simulink library "xpcobsoletelib"  (Simulink 6.0)
settings: Solver=ode45  SolverMode=SingleTasking  StartTime=0.0  StopTime=10.0  RelTol=1e-3
values from neighbouring files (symbols this model uses):
  channels = round(channels)    [mbwaudpmc.m]
undefined symbols (not defined in the file or in its folder): mdiobvmpmcdio64, menccbcioquad
settings Model: Creator=adowd  LastModifiedBy=adowd
settings DataIOCC: SignalLoggingName=logsOut
settings OptimizationCC: BooleanDataType=off
settings DebuggingCC: CheckExecutionContextPreStartOutputMsg=on  CheckExecutionContextRuntimeOutputMsg=on  SolverPrmCheckMsg=none
settings HardwareCC: TargetUnknown=on
settings GRTTargetCC: UtilityFuncGeneration=Automatic  LifeSpan=inf
settings SFSimCC: SFSimApplyToAllLibs=on  SFSimBuildMode=Incremental

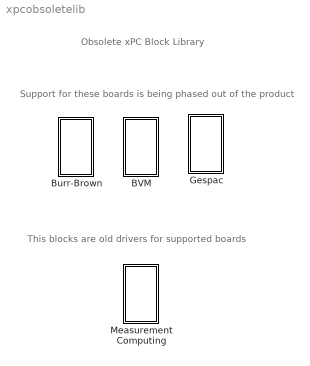
== system xpcobsoletelib ==
  note: Obsolete xPC Block Library
  note: Support for these boards is being phased out of the product
  note: This blocks are old drivers for supported boards
  BVM : Subsystem  EnableExecutionContextPropagation=on
  Burr-Brown : Subsystem  EnableExecutionContextPropagation=on
  Gespac : Subsystem  EnableExecutionContextPropagation=on
  Measurement Computing : Subsystem  EnableExecutionContextPropagation=on

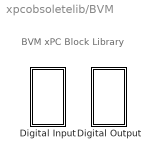
== system xpcobsoletelib/BVM ==
  note: BVM xPC Block Library
  Digital Input : Subsystem  EnableExecutionContextPropagation=on
  Digital Output : Subsystem  EnableExecutionContextPropagation=on

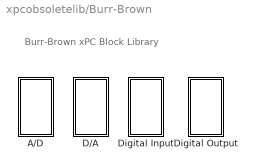
== system xpcobsoletelib/Burr-Brown ==
  note: Burr-Brown xPC Block Library
  A/D : Subsystem  EnableExecutionContextPropagation=on
  D/A : Subsystem  EnableExecutionContextPropagation=on
  Digital Input : Subsystem  EnableExecutionContextPropagation=on
  Digital Output : Subsystem  EnableExecutionContextPropagation=on

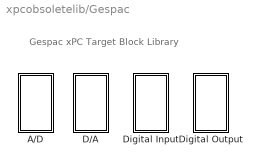
== system xpcobsoletelib/Gespac ==
  note: Gespac xPC Target Block Library
  A/D : Subsystem  EnableExecutionContextPropagation=on
  D/A : Subsystem  EnableExecutionContextPropagation=on
  Digital Input : Subsystem  EnableExecutionContextPropagation=on
  Digital Output : Subsystem  EnableExecutionContextPropagation=on

== system xpcobsoletelib/Measurement Computing ==
  note: Measurement Computing  xPC Target
      | Block Library (Obsolete)
  Incremental Encoder : Subsystem  EnableExecutionContextPropagation=on

== system xpcobsoletelib/BVM/Digital Input ==
  "PMCDIO64 " : S-Function  InitFcn=mdiobvmpmcdio64(1)  FunctionName=dibvmpmcdio64  Parameters=channel, port, ts, pcislot, config, fmt  mask(PMCDIO64-di){fmt=32 One bit channels, channel=[1], stopaction=, initial=, port=1, ts=0.001, pcislot=-1}
      mask prompts: fmt "Format:"; channel "Channel vector:"; port "Port (1-2):"; ts "Sample time:"; pcislot "PCI slot (-1: autosearch):"
      mask help:
      | PMCDIO64
      | BVM
      | Digital Input
      mask init:
      | [maskdisplay, maskdescription, config, initial, stopaction]=mdiobvmpmcdio64( 2, port, fmt, channel, stopaction, initial, pcislot); 
      | set_param(gcb,'MaskDisplay',maskdisplay);
      | set_param(gcb,'MaskDescription', maskdescription );
      mask Help: helpview(fullfile(docroot, 'mapfiles', 'xpc.map'), 'BVM_PMCDIO64_DIN')
      mask StyleString: popup(Single 32 bit port|32 One bit channels),edit,edit,edit,popup(1|2),edit,edit
      mask CallbackString:
      | maskvalues=get_param(gcb,'MaskValues');
      | 
      | fmt=maskvalues{1};
      | 
      | if fmt(1)=='3'
      | 
      | 	set_param(gcb, 'MaskEnables',{'on', 'on', 'off', 'off', 'on','on','on'});
      | 
      | else
      | 
      | 	set_param(gcb,'MaskEnables', {'on', 'off', 'off', 'off', 'on','on','on'});
      | 
      | end||||||
      mask Display: disp('PMCDIO64\nBVM\nDigital Input');port_label('output',1,'1');

== system xpcobsoletelib/BVM/Digital Output ==
  "PMCDIO64 1 " : S-Function  InitFcn=mdiobvmpmcdio64(1)  FunctionName=dobvmpmcdio64  Parameters=channel, port, ts, pcislot, config, fmt, stopaction, initial  mask(PMCDIO64-do){fmt=32 One bit channels, channel=[1], stopaction=[0], initial=[0], port=1, ts=0.001, pcislot=-1}
      mask prompts: fmt "Format:"; channel "Channel vector:"; stopaction "Reset action vector:"; initial "Initial value vector:"; port "Port (1-2):"; ts "Sample time:"; pcislot "PCI slot (-1: autosearch):"
      mask help:
      | PMCDIO64
      | BVM
      | Digital Output
      mask init:
      | [ maskdisplay, maskdescription, config, initial, stopaction ]=mdiobvmpmcdio64( 2, port, fmt, channel, stopaction, initial, pcislot);
      | set_param( gcb, 'MaskDisplay', maskdisplay );
      | set_param( gcb, 'MaskDescription', maskdescription );
      mask Help: helpview(fullfile(docroot, 'mapfiles', 'xpc.map'), 'BVM_PMCDIO64-1_DOUT')
      mask StyleString: popup(Single 32 bit port|32 One bit channels),edit,edit,edit,popup(1|2),edit,edit
      mask CallbackString:
      | maskvalues=get_param(gcb,'MaskValues');
      | 
      | fmt=maskvalues{1};
      | 
      | if fmt(1)=='3'
      | 
      | 	set_param(gcb, 'MaskEnables',{'on', 'on', 'on', 'on', 'on','on','on'});
      | 
      | else
      | 
      | 	set_param(gcb,'MaskEnables', {'on', 'off', 'on', 'on', 'on','on','on'});
      | 
      | end
      | 
      | ||||||
      mask Display: disp('PMCDIO64\nBVM\nDigital Output');port_label('input',1,'1');

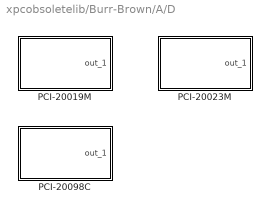
== system xpcobsoletelib/Burr-Brown/A/D ==
  "PCI-20019M " : Subsystem  EnableExecutionContextPropagation=on  mask(Analog Input Module){channels=1, range=-10, sampletime=0.001, module=1, baseaddress=0xd000}
      mask prompts: channels "Number of channels:"; range "Range vector:"; sampletime "Sample time:"; module "Module number (1-3):"; baseaddress "Base address (i.e. 0xd000):"
      mask help:
      | Burr-Brown
      | PCI-20019M
      | Analog Input
      mask init:
      | baseaddress=hex2dec(baseaddress(3:end));
      mask Help: helpview(fullfile(docroot, 'mapfiles', 'xpc.map'), 'Burr-Brown_PCI-20019M_AD')
      mask Display: disp('PCI-20019M\nBurr-Brown\nAnalog Input')
  "PCI-20023M " : Subsystem  EnableExecutionContextPropagation=on  mask(Analog Input Module){channels=1, range=-10, sampletime=0.001, module=1, baseaddress=0xd000}
      mask prompts: channels "Number of channels:"; range "Range vector:"; sampletime "Sample time:"; module "Module number (1-3):"; baseaddress "Base address (i.e. 0xd000):"
      mask help:
      | Burr-Brown
      | PCI-20023M
      | Analog Input
      mask init:
      | baseaddress=hex2dec(baseaddress(3:end));
      mask Help: helpview(fullfile(docroot, 'mapfiles', 'xpc.map'), 'Burr-Brown_PCI-20023M_AD')
      mask Display: disp('PCI-20023M\nBurr-Brown\nAnalog Input')
  "PCI-20098C " : Subsystem  EnableExecutionContextPropagation=on  mask(Analog Input Module){channels=1, range=+- 10 V, mux=Single-ended (16 channels), sampletime=0.001, baseaddress=0xd000}
      mask prompts: channels "Number of channels:"; range "Range vector:"; mux "Input coupling:"; sampletime "Sample time:"; baseaddress "Base address (i.e. 0xd000):"
      mask help:
      | Burr-Brown
      | PCI-20098C
      | Analog Input
      mask init:
      | baseaddress=hex2dec(baseaddress(3:end));
      mask Help: helpview(fullfile(docroot, 'mapfiles', 'xpc.map'), 'Burr-Brown_PCI-20098C_AD')
      mask StyleString: edit,popup(+- 10 V|+- 5V|0-10V),popup(Single-ended (16 channels)|Differential (8 channels)),edit,edit
      mask Display: disp('PCI-20098C\nBurr-Brown\nAnalog Input')

== system xpcobsoletelib/Burr-Brown/D/A ==
  "PCI-20003M " : Subsystem  EnableExecutionContextPropagation=on  mask(Analog Output Module){channels=[-10], sampletime=0.001, module=1, baseaddress=0xd000}
      mask prompts: channels "Channel vector:"; sampletime "Sample time:"; module "Module number (1-3):"; baseaddress "Base address (i.e. 0xd000):"
      mask help:
      | Burr-Brown
      | PCI-20003M
      | Analog Output
      mask init:
      | baseaddress=hex2dec(baseaddress(3:end));
      mask Help: helpview(fullfile(docroot, 'mapfiles', 'xpc.map'), 'Burr-Brown_PCI-20003M_DA')
      mask Display: disp('PCI-20003M\nBurr-Brown\nAnalog Output')

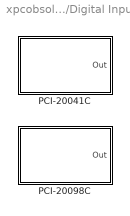
== system xpcobsoletelib/Burr-Brown/Digital Input ==
  "PCI-20041C " : Subsystem  EnableExecutionContextPropagation=on  mask(Digital Input Module){n_channels=1, port=0, sample_time=0.001, baseaddress=0xd000}
      mask prompts: n_channels "Number of channels:"; port "Port number (0-3):"; sample_time "Sample time:"; baseaddress "Base address (i.e. 0xd000):"
      mask help:
      | Burr Brown
      | PCI-20041C
      | Digital Input
      mask init:
      | baseaddress=hex2dec(baseaddress(3:end));
      mask Help: helpview(fullfile(docroot, 'mapfiles', 'xpc.map'), 'Burr-Brown_PCI-20041C_DIN')
      mask Display: disp('PCI-20041C\nBurr-Brown\nDigital Input')
  "PCI-20098C " : Subsystem  EnableExecutionContextPropagation=on  mask(Digital Input Module){n_channels=1, port=A, sample_time=0.001, baseaddress=0xd000}
      mask prompts: n_channels "Number of channels:"; sample_time "Sample time:"; baseaddress "Base address (i.e. 0xd000):"
      mask help:
      | Burr Brown
      | PCI-20098C
      | Digital Input
      mask init:
      | baseaddress=hex2dec(baseaddress(3:end));
      mask Help: helpview(fullfile(docroot, 'mapfiles', 'xpc.map'), 'Burr-Brown_PCI-20098C_DIN')
      mask StyleString: edit,popup(A|B),edit,edit
      mask Display: disp('PCI-20098C\nBurr-Brown\nDigital Input')

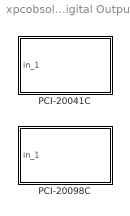
== system xpcobsoletelib/Burr-Brown/Digital Output ==
  "PCI-20041C " : Subsystem  EnableExecutionContextPropagation=on  mask(Digital Output Module){n_channels=1, port=0, sample_time=0.001, baseaddress=0xd000}
      mask prompts: n_channels "Number of channels:"; port "Port number (0-3):"; sample_time "Sample time:"; baseaddress "Base address (i.e. 0xd000):"
      mask help:
      | Burr Brown
      | PCI-20041C
      | Digital Output
      mask init:
      | baseaddress=hex2dec(baseaddress(3:end));
      mask Help: helpview(fullfile(docroot, 'mapfiles', 'xpc.map'), 'Burr-Brown_PCI-20041C_DOUT')
      mask Display: disp('PCI-20041C\nBurr-Brown\nDigital Output')
  "PCI-20098C " : Subsystem  EnableExecutionContextPropagation=on  mask(Digital Output Module){n_channels=1, port=A, sample_time=0.001, baseaddress=0xd000}
      mask prompts: n_channels "Number of channels:"; sample_time "Sample time:"; baseaddress "Base address (i.e. 0xd000):"
      mask help:
      | Burr Brown
      | PCI-20098C
      | Digital Output
      mask init:
      | baseaddress=hex2dec(baseaddress(3:end));
      mask Help: helpview(fullfile(docroot, 'mapfiles', 'xpc.map'), 'Burr-Brown_PCI-20098C_DOUT')
      mask StyleString: edit,popup(A|B),edit,edit
      mask Display: disp('PCI-20098C\nBurr-Brown\nDigital Output')

== system xpcobsoletelib/Gespac/A/D ==
  "GESADA-1 " : Subsystem  EnableExecutionContextPropagation=on  mask(Analog Input Module){channels=1, range=+-10 V, mux=Single-ended (16 channels), sampletime=0.001, baseaddress=0x300}
      mask prompts: channels "Number of channels:"; range "Range vector:"; mux "Input coupling:"; sampletime "Sample time:"; baseaddress "Base address (i.e. 0xd000):"
      mask help:
      | GESADA-1
      | Gespac
      | Analog Input
      mask init:
      | baseaddress=hex2dec(baseaddress(3:end));
      mask Help: helpview(fullfile(docroot, 'mapfiles', 'xpc.map'), 'Gespac_GESADA-1_AD')
      mask StyleString: edit,popup(+-10 V|+-5 V|0-10 V),popup(Single-ended (16 channels)|Differential (8 channels)),edit,edit
      mask Display: disp('GESADA-1\nGespac\nAnalog Input')

== system xpcobsoletelib/Gespac/D/A ==
  "GESADA-1 " : Subsystem  EnableExecutionContextPropagation=on  mask(Analog Output Module){channels=[-10], sampletime=0.001, baseaddress=0x300}
      mask prompts: channels "Channel vector:"; sampletime "Sample time:"; baseaddress "Base address (i.e. 0xd000):"
      mask help:
      | GESADA-1
      | Gespac
      | Analog Output
      mask init:
      | baseaddress=hex2dec(baseaddress(3:end));
      mask Help: helpview(fullfile(docroot, 'mapfiles', 'xpc.map'), 'Gespac_GESADA-1_DA')
      mask Display: disp('GESADA-1\nGespac\nAnalog Output')

== system xpcobsoletelib/Gespac/Digital Input ==
  "GESPIA-2A " : Subsystem  EnableExecutionContextPropagation=on  mask(Digital Input Module){n_channels=1, port=PIA0 A, sample_time=0.001, baseaddress=0x300}
      mask prompts: n_channels "Number of channels:"; port "Port name:"; sample_time "Sample time:"; baseaddress "Base address (i.e. 0xd000):"
      mask help:
      | Gespac
      | GESPIA-2A
      | Digital Input
      mask init:
      | baseaddress=hex2dec(baseaddress(3:end));
      mask Help: helpview(fullfile(docroot, 'mapfiles', 'xpc.map'), 'Gespac_GESPIA-2A_DIN')
      mask StyleString: edit,popup(PIA0 A|PIA0 B|PIA1 A|PIA1 B),edit,edit
      mask Display: disp('GESPIA-2A\nGespac\nDigital Input')

== system xpcobsoletelib/Gespac/Digital Output ==
  "GESPIA-2A " : Subsystem  EnableExecutionContextPropagation=on  mask(Digital Output Module){n_channels=1, port=PIA0 A, sample_time=0.001, baseaddress=0x300}
      mask prompts: n_channels "Number of channels:"; port "Port name:"; sample_time "Sample time:"; baseaddress "Base address (i.e. 0xd000):"
      mask help:
      | Gespac
      | GESPIA-2A
      | Digital Output
      mask init:
      | baseaddress=hex2dec(baseaddress(3:end));
      mask Help: helpview(fullfile(docroot, 'mapfiles', 'xpc.map'), 'Gespac_GESPIA-2A_DOUT')
      mask StyleString: edit,popup(PIA0 A|PIA0 B|PIA1 A|PIA1 B),edit,edit
      mask Display: disp('GESPIA-2A\nGespac\nDigital Output')

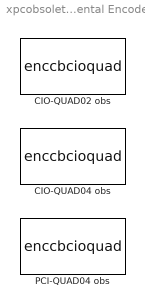
== system xpcobsoletelib/Measurement Computing/Incremental Encoder ==
  CIO-QUAD02 obs : S-Function  InitFcn=menccbcioquad(0);  FunctionName=enccbcioquad  Parameters=convBaseAddr, res, modetype, module, counting, rotation, prescale, ts, boardtype  mask(enccbcioquad){module=1, counting=Only First, rotation=Clockwise, modetype=single, res=1024, prescale=0, ts=0.001, baseAddr=0x300}
      mask prompts: module "Function module:"; counting "Counter reset by index:"; rotation "Positive rotation:"; modetype "Mode:"; res "Resolution:"; prescale "Filter prescale factor:"; ts "Sample time:"; baseAddr "Base address (i.e. 0xd000):"
      mask help:
      | CIO-QUAD02
      | Computer Boards
      | Incremental Encoder
      mask init:
      | convBaseAddr = 0;
      | boardtype = 1;
      | [convBaseAddr]=menccbcioquad(1, module ,baseAddr, 0, boardtype);
      mask Help: helpview(fullfile(docroot, 'mapfiles', 'xpc.map'), 'ComputerBoards_CIO-QUAD02_Encoder')
      mask StyleString: popup(1|2),popup(Continuous|Only first|Index input disabled),popup(Clockwise|Counter Clockwise),popup(Single|Double|Quadruple),edit,edit,edit,edit
      mask Display: text(0.05,0.75,'CIO-QUAD02','horizontalAlignment','left');text(0.05,0.5,'Comp. Boards','horizontalAlignment','left');text(0.05,0.25,'Inc. Encoder','horizontalAlignment','left');port_label('output',1,'Angle')port_label('output',2,'Turns')port_label('output',3,'Init')
  CIO-QUAD04 obs : S-Function  InitFcn=menccbcioquad(0);  FunctionName=enccbcioquad  Parameters=convBaseAddr, res, modetype, module, counting, rotation, prescale, ts, boardtype  mask(enccbcioquad){module=1, counting=Only first, rotation=Clockwise, modetype=Single, res=1024, prescale=0, ts=0.001, baseAddr=0x300}
      mask prompts: module "Function module:"; counting "Counting reset by index:"; rotation "Positive rotation:"; modetype "Mode:"; res "Resolution:"; prescale "Filter prescale factor:"; ts "Sample time:"; baseAddr "Base address (i.e. 0xd000):"
      mask help:
      | CIO-QUAD04
      | Computer Boards
      | Incremental Encoder
      mask init:
      | convBaseAddr = 0;
      | boardtype = 2;
      | [convBaseAddr]=menccbcioquad(1, module ,baseAddr, 0, boardtype);
      mask Help: helpview(fullfile(docroot, 'mapfiles', 'xpc.map'), 'ComputerBoards_CIO-QUAD04_Encoder')
      mask StyleString: popup(1|2|3|4),popup(Continuous|Only first|Index input disabled),popup(Clockwise|Counter Clockwise),popup(Single|Double|Quadruple),edit,edit,edit,edit
      mask Display: text(0.05,0.75,'CIO-QUAD04','horizontalAlignment','left');text(0.05,0.5,'Comp. Boards','horizontalAlignment','left');text(0.05,0.25,'Inc. Encoder','horizontalAlignment','left');port_label('output',1,'Angle')port_label('output',2,'Turns')port_label('output',3,'Init')
  PCI-QUAD04 obs : S-Function  InitFcn=menccbcioquad(0);  FunctionName=enccbcioquad  Parameters=convBaseAddr, res, modetype, module, counting, rotation, prescale, ts, boardtype  mask(enccbcioquad){module=1, counting=Only first, rotation=Clockwise, modetype=Single, res=1024, prescale=0, ts=0.001, convBaseAddr=-1}
      mask prompts: module "Function module:"; counting "Counting reset by index:"; rotation "Positive rotation:"; modetype "Mode:"; res "Resolution:"; prescale "Filter prescale factor:"; ts "Sample time:"; convBaseAddr "PCI slot (-1: autosearch):"
      mask help:
      | PCI-QUAD04
      | Computer Boards
      | Incremental Encoder
      mask init:
      | boardtype = 3;
      | menccbcioquad(1, module ,'0x300', convBaseAddr, boardtype);
      mask Help: helpview(fullfile(docroot, 'mapfiles', 'xpc.map'), 'ComputerBoards_PCI-QUAD04_Encoder')
      mask StyleString: popup(1|2|3|4),popup(Continuous|Only first|Index input disabled),popup(Clockwise|Counter Clockwise),popup(Single|Double|Quadruple),edit,edit,edit,edit
      mask Display: text(0.05,0.75,'PCI-QUAD04','horizontalAlignment','left');text(0.05,0.5,'Comp. Boards','horizontalAlignment','left');text(0.05,0.25,'Inc. Encoder','horizontalAlignment','left');port_label('output',1,'Angle')port_label('output',2,'Turns')port_label('output',3,'Init')

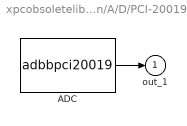
== system xpcobsoletelib/Burr-Brown/A/D/PCI-20019M  ==
  ADC : S-Function  FunctionName=adbbpci20019  Parameters=channels, range, sampletime, module, baseaddress
  out_1 : Outport  InitialOutput=0
  wires:
  ADC/1 -> out_1/1

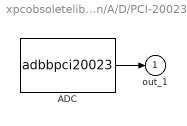
== system xpcobsoletelib/Burr-Brown/A/D/PCI-20023M  ==
  ADC : S-Function  FunctionName=adbbpci20023  Parameters=channels, range, sampletime, module, baseaddress
  out_1 : Outport  InitialOutput=0
  wires:
  ADC/1 -> out_1/1

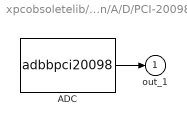
== system xpcobsoletelib/Burr-Brown/A/D/PCI-20098C  ==
  ADC : S-Function  FunctionName=adbbpci20098  Parameters=channels, range, mux, sampletime, baseaddress
  out_1 : Outport  InitialOutput=0
  wires:
  ADC/1 -> out_1/1

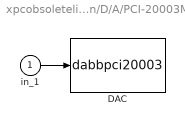
== system xpcobsoletelib/Burr-Brown/D/A/PCI-20003M  ==
  in_1 : Inport  LatchInput=off
  DAC : S-Function  FunctionName=dabbpci20003  Parameters=channels, sampletime, module, baseaddress
  wires:
  in_1/1 -> DAC/1

== system xpcobsoletelib/Burr-Brown/Digital Input/PCI-20041C  ==
  S-Function : S-Function  FunctionName=dibbpci20041  Parameters=n_channels,port,sample_time,baseaddress
  Out : Outport  InitialOutput=0
  wires:
  S-Function/1 -> Out/1

== system xpcobsoletelib/Burr-Brown/Digital Input/PCI-20098C  ==
  DAC : S-Function  FunctionName=dibbpci20098  Parameters=n_channels,port,sample_time,baseaddress
  Out : Outport  InitialOutput=0
  wires:
  DAC/1 -> Out/1

== system xpcobsoletelib/Burr-Brown/Digital Output/PCI-20041C  ==
  in_1 : Inport  LatchInput=off
  DAC : S-Function  FunctionName=dobbpci20041  Parameters=n_channels,port,sample_time,baseaddress
  wires:
  in_1/1 -> DAC/1

== system xpcobsoletelib/Burr-Brown/Digital Output/PCI-20098C  ==
  in_1 : Inport  LatchInput=off
  DAC : S-Function  FunctionName=dobbpci20098  Parameters=n_channels,port,sample_time,baseaddress
  wires:
  in_1/1 -> DAC/1

== system xpcobsoletelib/Gespac/A/D/GESADA-1  ==
  ADC : S-Function  FunctionName=adgesada1  Parameters=channels, range, mux, sampletime, baseaddress
  out_1 : Outport  InitialOutput=0
  wires:
  ADC/1 -> out_1/1

== system xpcobsoletelib/Gespac/D/A/GESADA-1  ==
  in_1 : Inport  LatchInput=off
  DAC : S-Function  FunctionName=dagesada1  Parameters=channels, sampletime, baseaddress
  wires:
  in_1/1 -> DAC/1

== system xpcobsoletelib/Gespac/Digital Input/GESPIA-2A  ==
  DAC1 : S-Function  FunctionName=digespia2a  Parameters=n_channels,port,sample_time,baseaddress
  out_1 : Outport  InitialOutput=0
  wires:
  DAC1/1 -> out_1/1

== system xpcobsoletelib/Gespac/Digital Output/GESPIA-2A  ==
  in_1 : Inport  LatchInput=off
  DAC : S-Function  FunctionName=dogespia2a  Parameters=n_channels,port,sample_time,baseaddress
  wires:
  in_1/1 -> DAC/1
